simulink model "lab2_4bmy"  (R2022a)
settings: Solver=ode3  StartTime=0.0  StopTime=Tmdl  FixedStep=To/100  RelTol=1e-3
values from neighbouring files (symbols this model uses):
  ob =     [data.mat]
undefined symbols (not defined in the file or in its folder): crl, spl, stl, To
libraries: fl_lib x22, nesl_utility x18
settings Model: Creator=osini  LastModifiedBy=sasha

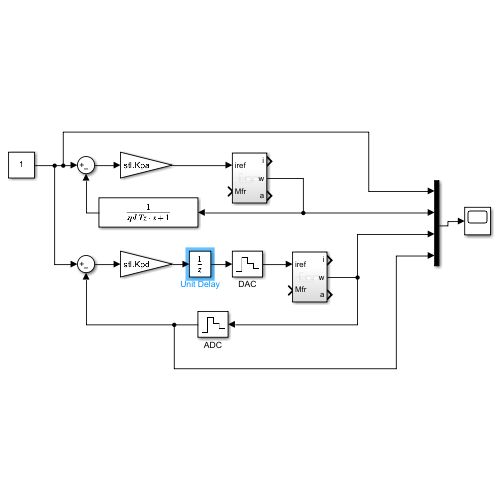
[thumbnail: Simulink's stored preview of the top-level diagram]
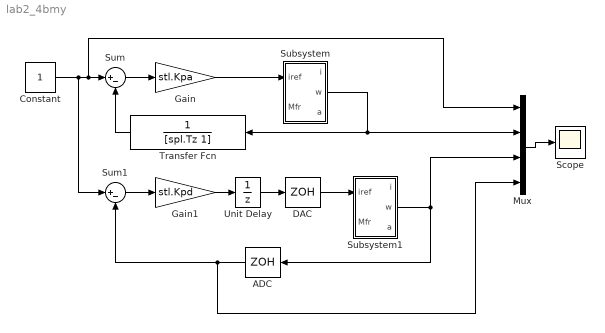
== system lab2_4bmy ==
  ADC : ZeroOrderHold  SampleTime=To
  Constant : Constant
  DAC : ZeroOrderHold  SampleTime=To
  Gain : Gain  Gain=stl.Kpa
  Gain1 : Gain  Gain=stl.Kpd
  Mux : Mux
  Scope : Scope
  Subsystem : Subsystem
  Subsystem1 : Subsystem
  Sum : Sum  Inputs=|+-
  Sum1 : Sum  Inputs=|+-
  Transfer Fcn : TransferFcn  Denominator=[spl.Tz 1]
  Unit Delay : UnitDelay  SampleTime=To  HasFrameUpgradeWarning=on
  wires:
  Sum/1 -> Gain/1
  Subsystem/2(w) -> Mux/2, Transfer Fcn/1
  Gain/1 -> Subsystem/1(iref)
  Subsystem1/2(w) -> Mux/3, ADC/1
  Sum1/1 -> Gain1/1
  Constant/1 -> Sum1/1, Mux/1, Sum/1
  Gain1/1 -> Unit Delay/1
  DAC/1 -> Subsystem1/1(iref)
  ADC/1 -> Mux/4, Sum1/2
  Mux/1 -> Scope/1
  Transfer Fcn/1 -> Sum/2
  Unit Delay/1 -> DAC/1

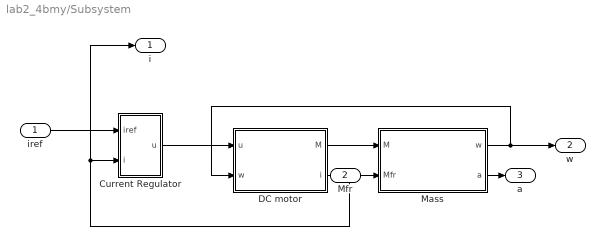
== system lab2_4bmy/Subsystem ==
  iref : Inport
  Mfr : Inport  Port=2
  Current Regulator : Subsystem
  DC motor : Subsystem
  Mass : Subsystem
  i : Outport
  w : Outport  Port=2
  a : Outport  Port=3
  wires:
  DC motor/1(M) -> Mass/1(M)
  Mass/1(w) -> w/1, DC motor/2(w)
  Mass/2(a) -> a/1
  DC motor/2(i) -> i/1, Current Regulator/2(i)
  Current Regulator/1(u) -> DC motor/1(u)
  iref/1 -> Current Regulator/1(iref)
  Mfr/1 -> Mass/2(Mfr)

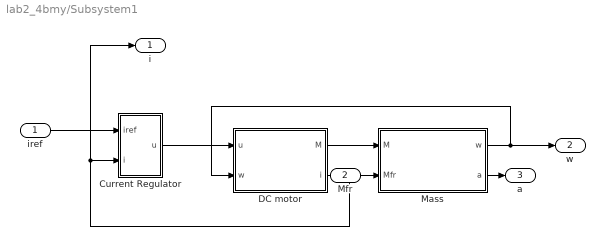
== system lab2_4bmy/Subsystem1 ==
  iref : Inport
  Mfr : Inport  Port=2
  Current Regulator : Subsystem
  DC motor : Subsystem
  Mass : Subsystem
  i : Outport
  w : Outport  Port=2
  a : Outport  Port=3
  wires:
  DC motor/1(M) -> Mass/1(M)
  Mass/1(w) -> w/1, DC motor/2(w)
  Mass/2(a) -> a/1
  DC motor/2(i) -> i/1, Current Regulator/2(i)
  Current Regulator/1(u) -> DC motor/1(u)
  iref/1 -> Current Regulator/1(iref)
  Mfr/1 -> Mass/2(Mfr)

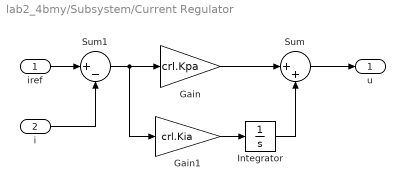
== system lab2_4bmy/Subsystem/Current Regulator ==
  iref : Inport
  i : Inport  Port=2
  Gain : Gain  Gain=crl.Kpa
  Gain1 : Gain  Gain=crl.Kia
  Integrator : Integrator
  Sum : Sum  Inputs=|++
  Sum1 : Sum  Inputs=|+-
  u : Outport
  wires:
  Sum/1 -> u/1
  Sum1/1 -> Gain/1, Gain1/1
  Integrator/1 -> Sum/2
  Gain/1 -> Sum/1
  Gain1/1 -> Integrator/1
  i/1 -> Sum1/2
  iref/1 -> Sum1/1

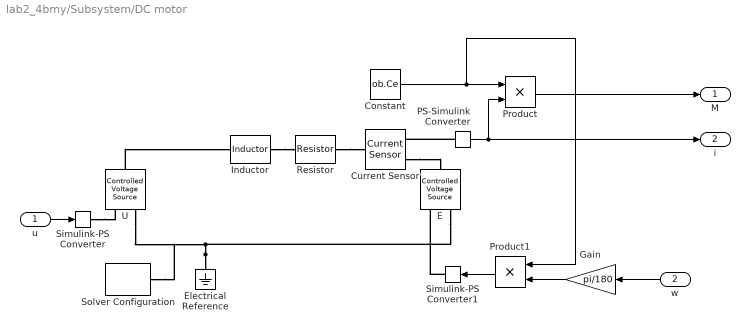
== system lab2_4bmy/Subsystem/DC motor ==
  u : Inport
  w : Inport  Port=2
  Constant : Constant  Value=ob.Ce
  Current Sensor : fl_lib/Electrical/Electrical Sensors/Current Sensor
      settings: SourceProductBaseCode=PW,SS,VE
  E : fl_lib/Electrical/Electrical Sources/Controlled Voltage Source
      settings: SourceProductBaseCode=PW,SS,VE
  Electrical Reference : fl_lib/Electrical/Electrical Elements/Electrical Reference
      settings: SourceProductBaseCode=PW,SS,VE
  Gain : Gain  Gain=pi/180
  Inductor : fl_lib/Electrical/Electrical Elements/Inductor  l=ob.L H  r=0 Ohm  g=1e-9 1/Ohm  i_specify=off  i_priority=None  i=0 A  i_nominal_specify=off  i_nominal_unit=A  i_nominal_value=1  v_specify=off  v_priority=None  v=0 V  v_nominal_specify=off  v_nominal_unit=V  v_nominal_value=1  i_L_specify=off  i_L_priority=High  i_L=0 A  i_L_nominal_specify=off  i_L_nominal_unit=A  i_L_nominal_value=1
      settings: SourceProductBaseCode=PW,SS,VE
  PS-Simulink Converter : nesl_utility/PS-Simulink Converter  PhysicalDomain=network_engine_domain  SubClassName=ps_output  LeftPortType=input  RightPortType=output  PseudoPeriodic=off  Frequencies=[]  VectorFormat=inherit  Unit=inherit  AffineConversion=off
      settings: SourceProductBaseCode=SS,PW,VE
  Product : Product
  Product1 : Product
  Resistor : fl_lib/Electrical/Electrical Elements/Resistor  R=ob.R Ohm  i_specify=off  i_priority=None  i=0 A  i_nominal_specify=off  i_nominal_unit=A  i_nominal_value=1  v_specify=off  v_priority=None  v=0 V  v_nominal_specify=off  v_nominal_unit=V  v_nominal_value=1
      settings: SourceProductBaseCode=PW,SS,VE
  Simulink-PS Converter : nesl_utility/Simulink-PS Converter  PhysicalDomain=network_engine_domain  SubClassName=ps_input  LeftPortType=input  RightPortType=output  PseudoPeriodic=off  Frequencies=[]  NoiseDistribution=none  NoiseParameters=[]  Unit=1  AffineConversion=off  FilteringAndDerivatives=provide  SimscapeFilterOrder=1  InputFilterTimeConstant=0.0001  UdotUserProvided=0
      settings: SourceProductBaseCode=SS,PW,VE
  Simulink-PS Converter1 : nesl_utility/Simulink-PS Converter  PhysicalDomain=network_engine_domain  SubClassName=ps_input  LeftPortType=input  RightPortType=output  PseudoPeriodic=off  Frequencies=[]  NoiseDistribution=none  NoiseParameters=[]  Unit=1  AffineConversion=off  FilteringAndDerivatives=provide  SimscapeFilterOrder=1  InputFilterTimeConstant=0.001  UdotUserProvided=0
      settings: SourceProductBaseCode=SS,PW,VE
  Solver Configuration : nesl_utility/Solver Configuration  PhysicalDomain=network_engine_domain  SubClassName=solver  LeftPortType=input  RightPortType=generic  Tones=[]  Harmonics=[]  SimulateNoise=off  Profile=off  UseLocalSampling=off  EnableSwitchedLinearOptims=on  FrequencyDomain=off  UseCCode=off  RelTol=0.001  AbsTol=0.001  MinStep=1e-09  ToWorkspace=off  RevertToSquareIcSolve=off  NumHomotopyIterations=100  PhasorMode=off  PhasorModeNumHarmonics=1  IndexReductionMethod=DerivativeReplacement  DoDC=off  ResidualTolerance=1e-09  UseLocalSolver=off  LocalSolverChoice=NE_BACKWARD_EULER_ADVANCER  LocalSolverSampleTime=0.001  DoFixedCost=off  MaxNonlinIter=3  MaxModeIter=2  ComputeImpulses=off  ImpulseIterations=2  LinearAlgebra=auto  LinearAlgebraNumThread=0  EquationFormulation=NE_TIME_EF  DelaysMemoryBudget=1024  AutomaticFiltering=on  FilteringTimeConstant=0.001  PartitionStorageMethod=AS_NEEDED  PartitionMemoryBudget=1024  PartitionMethod=ROBUST
      settings: SourceProductBaseCode=SS,PW,VE
  U : fl_lib/Electrical/Electrical Sources/Controlled Voltage Source
      settings: SourceProductBaseCode=PW,SS,VE
  M : Outport
  i : Outport  Port=2
  wires:
  PS-Simulink Converter/1 -> i/1, Product/2
  Constant/1 -> Product1/1, Product/1
  Product1/1 -> Simulink-PS Converter1/1
  Product/1 -> M/1
  u/1 -> Simulink-PS Converter/1
  w/1 -> Gain/1
  Gain/1 -> Product1/2
  connections:
  Electrical Reference/LConn1 -- Solver Configuration/RConn1 -- U/RConn2 -- E/RConn2
  PS-Simulink Converter/LConn1 -- Current Sensor/RConn1
  U/LConn1 -- Inductor/LConn1
  Resistor/RConn1 -- Current Sensor/LConn1
  Simulink-PS Converter1/RConn1 -- E/RConn1
  Current Sensor/RConn2 -- E/LConn1
  Simulink-PS Converter/RConn1 -- U/RConn1
  Inductor/RConn1 -- Resistor/LConn1

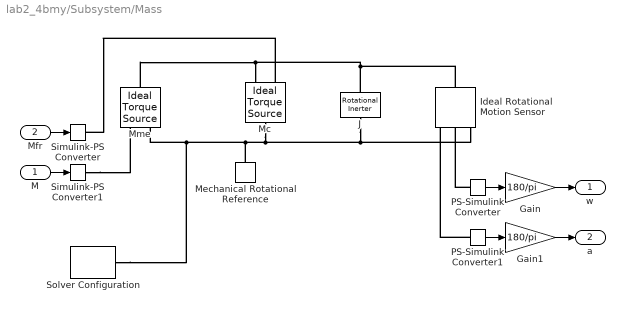
== system lab2_4bmy/Subsystem/Mass ==
  M : Inport
  Mfr : Inport  Port=2
  Gain : Gain  Gain=180/pi
  Gain1 : Gain  Gain=180/pi
  Ideal Rotational Motion Sensor : fl_lib/Mechanical/Mechanical Sensors/Ideal Rotational Motion Sensor  wrap_angle=simscape.enum.onoff.off  offset=0 rad
      settings: SourceProductBaseCode=PW,SS,VE
  J : fl_lib/Mechanical/Rotational Elements/Rotational Inerter  B=ob.J kg*m^2  w_specify=off  w_priority=High  w=0 rad/s  w_nominal_specify=off  w_nominal_unit=rad/s  w_nominal_value=1  t_specify=off  t_priority=None  t=0 N*m  t_nominal_specify=off  t_nominal_unit=N*m  t_nominal_value=1
      settings: SourceProductBaseCode=PW,SS,VE  InternalSimscapePortConfiguration="{\"Bottom\":[],\"Left\":[{\"id\":\"R\",\"label\":\"R\",\"type\":\"foundation.mechanical.rotational.rotational\"}],\"Right\":[{\"id\":\"C\",\"label\":\"C\",\"type\":\"foundation.mechanical.rotational.rotational\"}],\"Top\":[]}"
  Mc : fl_lib/Mechanical/Mechanical Sources/Ideal Torque Source
      settings: SourceProductBaseCode=PW,SS,VE
  Mechanical Rotational Reference : fl_lib/Mechanical/Rotational Elements/Mechanical Rotational Reference
      settings: SourceProductBaseCode=PW,SS,VE
  Mme : fl_lib/Mechanical/Mechanical Sources/Ideal Torque Source
      settings: SourceProductBaseCode=PW,SS,VE
  PS-Simulink Converter : nesl_utility/PS-Simulink Converter  PhysicalDomain=network_engine_domain  SubClassName=ps_output  LeftPortType=input  RightPortType=output  PseudoPeriodic=off  Frequencies=[]  VectorFormat=inherit  Unit=inherit  AffineConversion=off
      settings: SourceProductBaseCode=SS,PW,VE
  PS-Simulink Converter1 : nesl_utility/PS-Simulink Converter  PhysicalDomain=network_engine_domain  SubClassName=ps_output  LeftPortType=input  RightPortType=output  PseudoPeriodic=off  Frequencies=[]  VectorFormat=inherit  Unit=inherit  AffineConversion=off
      settings: SourceProductBaseCode=SS,PW,VE
  Simulink-PS Converter : nesl_utility/Simulink-PS Converter  PhysicalDomain=network_engine_domain  SubClassName=ps_input  LeftPortType=input  RightPortType=output  PseudoPeriodic=off  Frequencies=[]  NoiseDistribution=none  NoiseParameters=[]  Unit=1  AffineConversion=off  FilteringAndDerivatives=provide  SimscapeFilterOrder=1  InputFilterTimeConstant=0.001  UdotUserProvided=0
      settings: SourceProductBaseCode=SS,PW,VE
  Simulink-PS Converter1 : nesl_utility/Simulink-PS Converter  PhysicalDomain=network_engine_domain  SubClassName=ps_input  LeftPortType=input  RightPortType=output  PseudoPeriodic=off  Frequencies=[]  NoiseDistribution=none  NoiseParameters=[]  Unit=1  AffineConversion=off  FilteringAndDerivatives=provide  SimscapeFilterOrder=1  InputFilterTimeConstant=0.001  UdotUserProvided=0
      settings: SourceProductBaseCode=SS,PW,VE
  Solver Configuration : nesl_utility/Solver Configuration  PhysicalDomain=network_engine_domain  SubClassName=solver  LeftPortType=input  RightPortType=generic  Tones=[]  Harmonics=[]  SimulateNoise=off  Profile=off  UseLocalSampling=off  EnableSwitchedLinearOptims=on  FrequencyDomain=off  UseCCode=off  RelTol=0.001  AbsTol=0.001  MinStep=1e-09  ToWorkspace=off  RevertToSquareIcSolve=off  NumHomotopyIterations=100  PhasorMode=off  PhasorModeNumHarmonics=1  IndexReductionMethod=DerivativeReplacement  DoDC=off  ResidualTolerance=1e-09  UseLocalSolver=off  LocalSolverChoice=NE_BACKWARD_EULER_ADVANCER  LocalSolverSampleTime=0.001  DoFixedCost=off  MaxNonlinIter=3  MaxModeIter=2  ComputeImpulses=off  ImpulseIterations=2  LinearAlgebra=auto  LinearAlgebraNumThread=0  EquationFormulation=NE_TIME_EF  DelaysMemoryBudget=1024  AutomaticFiltering=on  FilteringTimeConstant=0.001  PartitionStorageMethod=AS_NEEDED  PartitionMemoryBudget=1024  PartitionMethod=ROBUST
      settings: SourceProductBaseCode=SS,PW,VE
  w : Outport
  a : Outport  Port=2
  wires:
  Mfr/1 -> Simulink-PS Converter/1
  M/1 -> Simulink-PS Converter1/1
  PS-Simulink Converter/1 -> Gain/1
  PS-Simulink Converter1/1 -> Gain1/1
  Gain/1 -> w/1
  Gain1/1 -> a/1
  connections:
  J/RConn1 -- Ideal Rotational Motion Sensor/RConn1 -- Mc/LConn1 -- Mechanical Rotational Reference/LConn1 -- Solver Configuration/RConn1 -- Mme/RConn2
  J/LConn1 -- Ideal Rotational Motion Sensor/LConn1 -- Mme/LConn1 -- Mc/RConn2
  PS-Simulink Converter/LConn1 -- Ideal Rotational Motion Sensor/RConn2
  PS-Simulink Converter1/LConn1 -- Ideal Rotational Motion Sensor/RConn3
  Simulink-PS Converter1/RConn1 -- Mme/RConn1
  Mc/RConn1 -- Simulink-PS Converter/RConn1

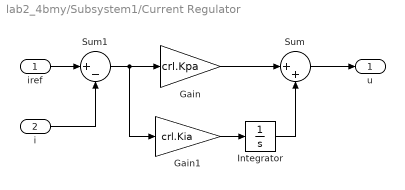
== system lab2_4bmy/Subsystem1/Current Regulator ==
  iref : Inport
  i : Inport  Port=2
  Gain : Gain  Gain=crl.Kpa
  Gain1 : Gain  Gain=crl.Kia
  Integrator : Integrator
  Sum : Sum  Inputs=|++
  Sum1 : Sum  Inputs=|+-
  u : Outport
  wires:
  Sum/1 -> u/1
  Sum1/1 -> Gain/1, Gain1/1
  Integrator/1 -> Sum/2
  Gain/1 -> Sum/1
  Gain1/1 -> Integrator/1
  i/1 -> Sum1/2
  iref/1 -> Sum1/1

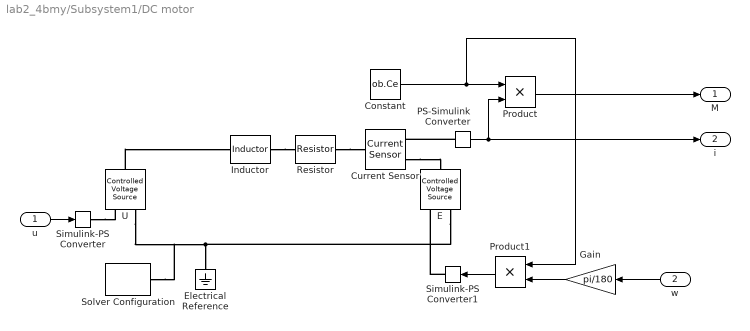
== system lab2_4bmy/Subsystem1/DC motor ==
  u : Inport
  w : Inport  Port=2
  Constant : Constant  Value=ob.Ce
  Current Sensor : fl_lib/Electrical/Electrical Sensors/Current Sensor
      settings: SourceProductBaseCode=PW,SS,VE
  E : fl_lib/Electrical/Electrical Sources/Controlled Voltage Source
      settings: SourceProductBaseCode=PW,SS,VE
  Electrical Reference : fl_lib/Electrical/Electrical Elements/Electrical Reference
      settings: SourceProductBaseCode=PW,SS,VE
  Gain : Gain  Gain=pi/180
  Inductor : fl_lib/Electrical/Electrical Elements/Inductor  l=ob.L H  r=0 Ohm  g=1e-9 1/Ohm  i_specify=off  i_priority=None  i=0 A  i_nominal_specify=off  i_nominal_unit=A  i_nominal_value=1  v_specify=off  v_priority=None  v=0 V  v_nominal_specify=off  v_nominal_unit=V  v_nominal_value=1  i_L_specify=off  i_L_priority=High  i_L=0 A  i_L_nominal_specify=off  i_L_nominal_unit=A  i_L_nominal_value=1
      settings: SourceProductBaseCode=PW,SS,VE
  PS-Simulink Converter : nesl_utility/PS-Simulink Converter  PhysicalDomain=network_engine_domain  SubClassName=ps_output  LeftPortType=input  RightPortType=output  PseudoPeriodic=off  Frequencies=[]  VectorFormat=inherit  Unit=inherit  AffineConversion=off
      settings: SourceProductBaseCode=SS,PW,VE
  Product : Product
  Product1 : Product
  Resistor : fl_lib/Electrical/Electrical Elements/Resistor  R=ob.R Ohm  i_specify=off  i_priority=None  i=0 A  i_nominal_specify=off  i_nominal_unit=A  i_nominal_value=1  v_specify=off  v_priority=None  v=0 V  v_nominal_specify=off  v_nominal_unit=V  v_nominal_value=1
      settings: SourceProductBaseCode=PW,SS,VE
  Simulink-PS Converter : nesl_utility/Simulink-PS Converter  PhysicalDomain=network_engine_domain  SubClassName=ps_input  LeftPortType=input  RightPortType=output  PseudoPeriodic=off  Frequencies=[]  NoiseDistribution=none  NoiseParameters=[]  Unit=1  AffineConversion=off  FilteringAndDerivatives=provide  SimscapeFilterOrder=1  InputFilterTimeConstant=0.001  UdotUserProvided=0
      settings: SourceProductBaseCode=SS,PW,VE
  Simulink-PS Converter1 : nesl_utility/Simulink-PS Converter  PhysicalDomain=network_engine_domain  SubClassName=ps_input  LeftPortType=input  RightPortType=output  PseudoPeriodic=off  Frequencies=[]  NoiseDistribution=none  NoiseParameters=[]  Unit=1  AffineConversion=off  FilteringAndDerivatives=provide  SimscapeFilterOrder=1  InputFilterTimeConstant=0.001  UdotUserProvided=0
      settings: SourceProductBaseCode=SS,PW,VE
  Solver Configuration : nesl_utility/Solver Configuration  PhysicalDomain=network_engine_domain  SubClassName=solver  LeftPortType=input  RightPortType=generic  Tones=[]  Harmonics=[]  SimulateNoise=off  Profile=off  UseLocalSampling=off  EnableSwitchedLinearOptims=on  FrequencyDomain=off  UseCCode=off  RelTol=0.001  AbsTol=0.001  MinStep=1e-09  ToWorkspace=off  RevertToSquareIcSolve=off  NumHomotopyIterations=100  PhasorMode=off  PhasorModeNumHarmonics=1  IndexReductionMethod=DerivativeReplacement  DoDC=off  ResidualTolerance=1e-09  UseLocalSolver=off  LocalSolverChoice=NE_BACKWARD_EULER_ADVANCER  LocalSolverSampleTime=0.001  DoFixedCost=off  MaxNonlinIter=3  MaxModeIter=2  ComputeImpulses=off  ImpulseIterations=2  LinearAlgebra=auto  LinearAlgebraNumThread=0  EquationFormulation=NE_TIME_EF  DelaysMemoryBudget=1024  AutomaticFiltering=on  FilteringTimeConstant=0.001  PartitionStorageMethod=AS_NEEDED  PartitionMemoryBudget=1024  PartitionMethod=ROBUST
      settings: SourceProductBaseCode=SS,PW,VE
  U : fl_lib/Electrical/Electrical Sources/Controlled Voltage Source
      settings: SourceProductBaseCode=PW,SS,VE
  M : Outport
  i : Outport  Port=2
  wires:
  PS-Simulink Converter/1 -> i/1, Product/2
  Constant/1 -> Product1/1, Product/1
  Product1/1 -> Simulink-PS Converter1/1
  Product/1 -> M/1
  u/1 -> Simulink-PS Converter/1
  w/1 -> Gain/1
  Gain/1 -> Product1/2
  connections:
  E/RConn2 -- Electrical Reference/LConn1 -- U/RConn2 -- Solver Configuration/RConn1
  PS-Simulink Converter/LConn1 -- Current Sensor/RConn1
  U/LConn1 -- Inductor/LConn1
  Resistor/RConn1 -- Current Sensor/LConn1
  Simulink-PS Converter1/RConn1 -- E/RConn1
  Current Sensor/RConn2 -- E/LConn1
  Simulink-PS Converter/RConn1 -- U/RConn1
  Inductor/RConn1 -- Resistor/LConn1

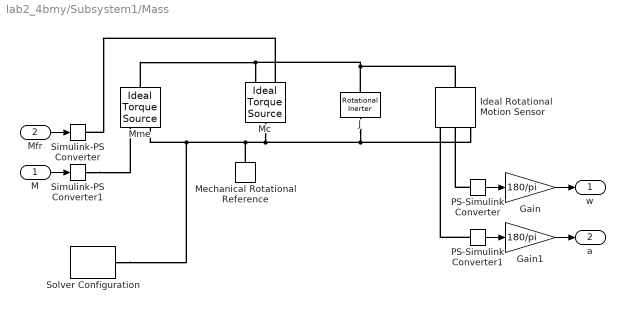
== system lab2_4bmy/Subsystem1/Mass ==
  M : Inport
  Mfr : Inport  Port=2
  Gain : Gain  Gain=180/pi
  Gain1 : Gain  Gain=180/pi
  Ideal Rotational Motion Sensor : fl_lib/Mechanical/Mechanical Sensors/Ideal Rotational Motion Sensor  wrap_angle=simscape.enum.onoff.off  offset=0 rad
      settings: SourceProductBaseCode=PW,SS,VE
  J : fl_lib/Mechanical/Rotational Elements/Rotational Inerter  B=ob.J kg*m^2  w_specify=off  w_priority=High  w=0 rad/s  w_nominal_specify=off  w_nominal_unit=rad/s  w_nominal_value=1  t_specify=off  t_priority=None  t=0 N*m  t_nominal_specify=off  t_nominal_unit=N*m  t_nominal_value=1
      settings: SourceProductBaseCode=PW,SS,VE  InternalSimscapePortConfiguration="{\"Bottom\":[],\"Left\":[{\"id\":\"R\",\"label\":\"R\",\"type\":\"foundation.mechanical.rotational.rotational\"}],\"Right\":[{\"id\":\"C\",\"label\":\"C\",\"type\":\"foundation.mechanical.rotational.rotational\"}],\"Top\":[]}"
  Mc : fl_lib/Mechanical/Mechanical Sources/Ideal Torque Source
      settings: SourceProductBaseCode=PW,SS,VE
  Mechanical Rotational Reference : fl_lib/Mechanical/Rotational Elements/Mechanical Rotational Reference
      settings: SourceProductBaseCode=PW,SS,VE
  Mme : fl_lib/Mechanical/Mechanical Sources/Ideal Torque Source
      settings: SourceProductBaseCode=PW,SS,VE
  PS-Simulink Converter : nesl_utility/PS-Simulink Converter  PhysicalDomain=network_engine_domain  SubClassName=ps_output  LeftPortType=input  RightPortType=output  PseudoPeriodic=off  Frequencies=[]  VectorFormat=inherit  Unit=inherit  AffineConversion=off
      settings: SourceProductBaseCode=SS,PW,VE
  PS-Simulink Converter1 : nesl_utility/PS-Simulink Converter  PhysicalDomain=network_engine_domain  SubClassName=ps_output  LeftPortType=input  RightPortType=output  PseudoPeriodic=off  Frequencies=[]  VectorFormat=inherit  Unit=inherit  AffineConversion=off
      settings: SourceProductBaseCode=SS,PW,VE
  Simulink-PS Converter : nesl_utility/Simulink-PS Converter  PhysicalDomain=network_engine_domain  SubClassName=ps_input  LeftPortType=input  RightPortType=output  PseudoPeriodic=off  Frequencies=[]  NoiseDistribution=none  NoiseParameters=[]  Unit=1  AffineConversion=off  FilteringAndDerivatives=provide  SimscapeFilterOrder=1  InputFilterTimeConstant=0.001  UdotUserProvided=0
      settings: SourceProductBaseCode=SS,PW,VE
  Simulink-PS Converter1 : nesl_utility/Simulink-PS Converter  PhysicalDomain=network_engine_domain  SubClassName=ps_input  LeftPortType=input  RightPortType=output  PseudoPeriodic=off  Frequencies=[]  NoiseDistribution=none  NoiseParameters=[]  Unit=1  AffineConversion=off  FilteringAndDerivatives=provide  SimscapeFilterOrder=1  InputFilterTimeConstant=0.001  UdotUserProvided=0
      settings: SourceProductBaseCode=SS,PW,VE
  Solver Configuration : nesl_utility/Solver Configuration  PhysicalDomain=network_engine_domain  SubClassName=solver  LeftPortType=input  RightPortType=generic  Tones=[]  Harmonics=[]  SimulateNoise=off  Profile=off  UseLocalSampling=off  EnableSwitchedLinearOptims=on  FrequencyDomain=off  UseCCode=off  RelTol=0.001  AbsTol=0.001  MinStep=1e-09  ToWorkspace=off  RevertToSquareIcSolve=off  NumHomotopyIterations=100  PhasorMode=off  PhasorModeNumHarmonics=1  IndexReductionMethod=DerivativeReplacement  DoDC=off  ResidualTolerance=1e-09  UseLocalSolver=off  LocalSolverChoice=NE_BACKWARD_EULER_ADVANCER  LocalSolverSampleTime=0.001  DoFixedCost=off  MaxNonlinIter=3  MaxModeIter=2  ComputeImpulses=off  ImpulseIterations=2  LinearAlgebra=auto  LinearAlgebraNumThread=0  EquationFormulation=NE_TIME_EF  DelaysMemoryBudget=1024  AutomaticFiltering=on  FilteringTimeConstant=0.001  PartitionStorageMethod=AS_NEEDED  PartitionMemoryBudget=1024  PartitionMethod=ROBUST
      settings: SourceProductBaseCode=SS,PW,VE
  w : Outport
  a : Outport  Port=2
  wires:
  Mfr/1 -> Simulink-PS Converter/1
  M/1 -> Simulink-PS Converter1/1
  PS-Simulink Converter/1 -> Gain/1
  PS-Simulink Converter1/1 -> Gain1/1
  Gain/1 -> w/1
  Gain1/1 -> a/1
  connections:
  Mme/RConn2 -- Mechanical Rotational Reference/LConn1 -- Ideal Rotational Motion Sensor/RConn1 -- J/RConn1 -- Mc/LConn1 -- Solver Configuration/RConn1
  Mme/LConn1 -- Mc/RConn2 -- J/LConn1 -- Ideal Rotational Motion Sensor/LConn1
  PS-Simulink Converter/LConn1 -- Ideal Rotational Motion Sensor/RConn2
  PS-Simulink Converter1/LConn1 -- Ideal Rotational Motion Sensor/RConn3
  Simulink-PS Converter1/RConn1 -- Mme/RConn1
  Mc/RConn1 -- Simulink-PS Converter/RConn1
